simulink model "radiation_test"  (Simulink 6.1)
settings: Solver=ode45  StartTime=0.0  StopTime=10.0  RelTol=1e-3
undefined symbols (not defined in the file): I, Radiation, radiation_lib
libraries: Accessories_lib x5, exposed_area_lib x2
settings Model: Creator=yliu03  LastModifiedBy=Dan T  ExtModeAutoUpdateStatusClock=off
settings DataIOCC: SignalLoggingName=sigsOut
settings HardwareCC: TargetUnknown=on

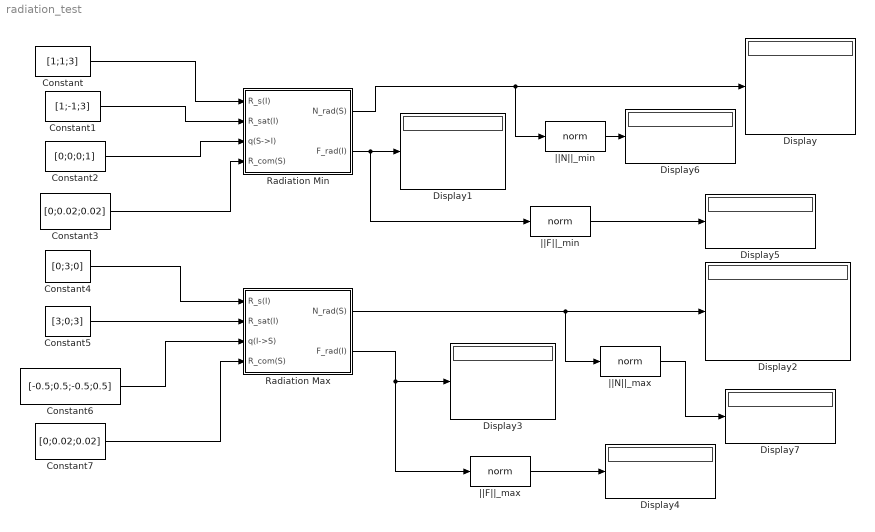
== system radiation_test ==
  Constant : Constant  Value=[1;1;3]
  Constant1 : Constant  Value=[1;-1;3]
  Constant2 : Constant  Value=[0;0;0;1]
  Constant3 : Constant  Value=[0;0.02;0.02]
  Constant4 : Constant  Value=[0;3;0]
  Constant5 : Constant  Value=[3;0;3]
  Constant6 : Constant  Value=[-0.5;0.5;-0.5;0.5]
  Constant7 : Constant  Value=[0;0.02;0.02]
  Display{,1..7} (8 alike) : Display
  Radiation Max : Subsystem  AncestorBlock=radiation_lib/Radiation (I)
  Radiation Min : Subsystem  AncestorBlock=radiation_lib/Radiation (I)
  ||F||_max : MATLABFcn  MATLABFcn=norm
  "||F||_min " : MATLABFcn  MATLABFcn=norm
  ||N||_max : MATLABFcn  MATLABFcn=norm
  ||N||_min : MATLABFcn  MATLABFcn=norm
  wires:
  Radiation Min/1(N_rad(S)) -> Display/1, ||N||_min/1
  Radiation Min/2(F_rad(I)) -> Display1/1, "||F||_min "/1
  Constant/1 -> Radiation Min/1(R_s(I))
  Constant1/1 -> Radiation Min/2(R_sat(I))
  Constant2/1 -> Radiation Min/3(q(S->I))
  Constant3/1 -> Radiation Min/4(R_com(S))
  Constant4/1 -> Radiation Max/1(R_s(I))
  Constant5/1 -> Radiation Max/2(R_sat(I))
  Constant7/1 -> Radiation Max/4(R_com(S))
  Constant6/1 -> Radiation Max/3(q(I->S))
  Radiation Max/1(N_rad(S)) -> Display2/1, ||N||_max/1
  Radiation Max/2(F_rad(I)) -> Display3/1, ||F||_max/1
  ||F||_max/1 -> Display4/1
  "||F||_min "/1 -> Display5/1
  ||N||_min/1 -> Display6/1
  ||N||_max/1 -> Display7/1

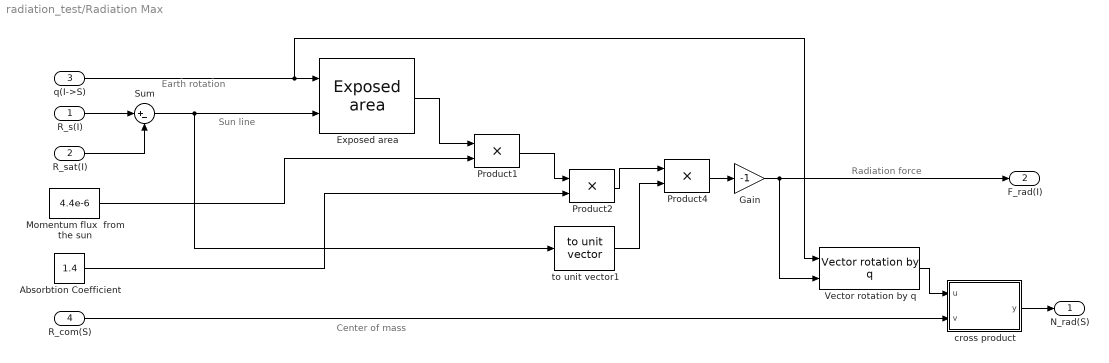
== system radiation_test/Radiation Max ==
  note: Radiation force
  note: Center of mass
  note: Earth rotation
  note: Sun line
  R_s(I) : Inport  Port=1  LatchInput=off
  R_sat(I) : Inport  Port=2  LatchInput=off
  q(I->S) : Inport  Port=3  LatchInput=off
  R_com(S) : Inport  Port=4  LatchInput=off
  Absorbtion Coefficient : Constant  Value=1.4
  Exposed area : exposed_area_lib/Exposed area
  Gain : Gain  Gain=-1  SaturateOnIntegerOverflow=on
  Momentum flux  from the sun : Constant  Value=4.4e-6
  Product1 : Product  SaturateOnIntegerOverflow=on
  Product2 : Product  SaturateOnIntegerOverflow=on
  Product4 : Product  SaturateOnIntegerOverflow=on
  Sum : Sum  Inputs=|+-  SaturateOnIntegerOverflow=on
  Vector rotation by q : Accessories_lib/Math utilities/Vector operations/Vector rotation by q
  cross product : Stateflow chart
  to unit vector1 : Accessories_lib/Math utilities/Vector operations/to unit vector
  N_rad(S) : Outport
  F_rad(I) : Outport  Port=2
  wires:
  Vector rotation by q/1 -> cross product/1(u)
  R_com(S)/1 -> cross product/2(v)
  Gain/1 -> F_rad(I)/1, Vector rotation by q/2
  Product4/1 -> Gain/1
  to unit vector1/1 -> Product4/2
  Product2/1 -> Product4/1
  Absorbtion Coefficient/1 -> Product2/2
  Product1/1 -> Product2/1
  Exposed area/1 -> Product1/1
  Momentum flux  from the sun/1 -> Product1/2
  Sum/1 -> Exposed area/2, to unit vector1/1
  q(I->S)/1 -> Vector rotation by q/1, Exposed area/1
  R_sat(I)/1 -> Sum/2
  R_s(I)/1 -> Sum/1
  cross product/1(y) -> N_rad(S)/1

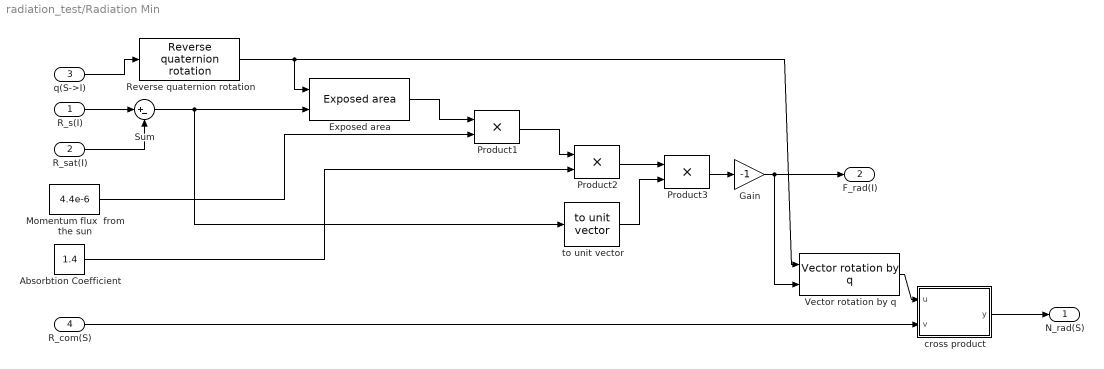
== system radiation_test/Radiation Min ==
  R_s(I) : Inport  Port=1  LatchInput=off
  R_sat(I) : Inport  Port=2  LatchInput=off
  q(S->I) : Inport  Port=3  LatchInput=off
  R_com(S) : Inport  Port=4  LatchInput=off
  Absorbtion Coefficient : Constant  Value=1.4
  Exposed area : exposed_area_lib/Exposed area
  Gain : Gain  Gain=-1  SaturateOnIntegerOverflow=on
  Momentum flux  from the sun : Constant  Value=4.4e-6
  Product1 : Product  SaturateOnIntegerOverflow=on
  Product2 : Product  SaturateOnIntegerOverflow=on
  "Product3 " : Product  SaturateOnIntegerOverflow=on
  Reverse quaternion rotation : Accessories_lib/Math utilities/Quaternion operations/Reverse quaternion rotation
  Sum : Sum  Inputs=|+-  SaturateOnIntegerOverflow=on
  Vector rotation by q : Accessories_lib/Math utilities/Vector operations/Vector rotation by q
  cross product : Stateflow chart
  to unit vector : Accessories_lib/Math utilities/Vector operations/to unit vector
  N_rad(S) : Outport
  F_rad(I) : Outport  Port=2
  wires:
  cross product/1(y) -> N_rad(S)/1
  Vector rotation by q/1 -> cross product/1(u)
  R_com(S)/1 -> cross product/2(v)
  Gain/1 -> F_rad(I)/1, Vector rotation by q/2
  "Product3 "/1 -> Gain/1
  to unit vector/1 -> "Product3 "/2
  Product2/1 -> "Product3 "/1
  Absorbtion Coefficient/1 -> Product2/2
  Product1/1 -> Product2/1
  Exposed area/1 -> Product1/1
  Momentum flux  from the sun/1 -> Product1/2
  Sum/1 -> to unit vector/1, Exposed area/2
  Reverse quaternion rotation/1 -> Vector rotation by q/1, Exposed area/1
  q(S->I)/1 -> Reverse quaternion rotation/1
  R_sat(I)/1 -> Sum/2
  R_s(I)/1 -> Sum/1

== matlab function Radiation Min/cross product ==
  data: u input inherited; y output inherited; v input inherited
function y = crossproduct(u,v)
% This block supports an embeddable subset of the MATLAB language.
% See the help menu for details. 

y = [u(2)*v(3)-u(3)*v(2);u(3)*v(1)-u(1)*v(3);u(1)*v(2)-u(2)*v(1)];

== matlab function Radiation Max/cross product ==
  data: u input inherited; y output inherited; v input inherited
function y = crossproduct(u,v)
% This block supports an embeddable subset of the MATLAB language.
% See the help menu for details. 

y = [u(2)*v(3)-u(3)*v(2);u(3)*v(1)-u(1)*v(3);u(1)*v(2)-u(2)*v(1)];
